simulink model "model_based_imp_ctrl_R2017b"  (Simulink 9.0)
settings: Solver=VariableStepAuto  StartTime=0.0  StopTime=60  FixedStep=0.00040  RelTol=1e-4  AbsTol=1e-7
values from neighbouring files (symbols this model uses):
  alpha = pi/180 * 13.6    (= 0.237364778271)    [IdealParameter.m]    (also in ParLuk11.m = deg2rad(13.6); Parameter.m = [-alpha_i;alpha_i;-alpha_i;alpha_i;-alpha_i;alpha_i]; ParameterIdeal.m = [-alpha_i;alpha_i;-alpha_i;alpha_i;-alpha_i;alpha_i]; ParameterVIVE.m = [alpha_i;-alpha_i;alpha_i;-alpha_i;alpha_i;-alpha_i])
  alpha_0 = alpha    (= 0.237364778271)    [IdealParameter.m]    (also in Parameter.m = alpha; ParameterIdeal.m = alpha*1.01; ParameterVIVE.m = alpha*1.01; ParameterVO.m = alpha*1.01)
  angular_noise = 0    [IdealParameter.m]    (also in Parameter.m = 0.5; ParameterIdeal.m; ParameterVIVE.m; ParameterVO.m)
  b = 1.1e-06    [IdealParameter.m]    (also in ParLuk11.m = 1.14e-07; Parameter.m = 8.944e-07; ParameterIdeal.m; ParameterVIVE.m)
  b_0 = b*1.15    (= 1.265e-06)    [IdealParameter.m]    (also in Parameter.m = 8.944e-07; ParameterIdeal.m; ParameterVIVE.m; ParameterVO.m)
  beta = 0    [IdealParameter.m]    (also in ParLuk11.m; Parameter.m = [beta_i; beta_i; beta_i; beta_i; beta_i; beta_i]; ParameterIdeal.m = [beta_i; beta_i; beta_i; beta_i; beta_i; beta_i]; ParameterVIVE.m = [beta_i; beta_i; beta_i; beta_i; beta_i; beta_i])
  beta_0 = beta    (= 0)    [IdealParameter.m]    (also in Parameter.m = beta; ParameterIdeal.m = beta*0.99; ParameterVIVE.m = beta*0.99; ParameterVO.m = beta*0.99)
  deltah = -0.0427    [Parameter.m]    (also in ParameterIdeal.m; ParameterVIVE.m = 0; ParameterVO.m; Parameter_old.m)
  deltah_0 = deltah    (= -0.0427)    [Parameter.m]    (also in ParameterIdeal.m = -0.041419; ParameterVIVE.m = 0; ParameterVO.m = -0.041419; Parameter_old.m = -0.041419)
  eta_rot = 50    [IdealParameter.m]    (also in Parameter.m = 2; ParameterIdeal.m = 20; ParameterVIVE.m = 5; ParameterVO.m = 2)
  g = 9.81    [IdealParameter.m]    (also in ParLuk11.m; Parameter.m; ParameterIdeal.m; ParameterVIVE.m)
  g_0 = g*0.99    (= 9.7119)    [IdealParameter.m]    (also in Parameter.m = 9.81; ParameterIdeal.m = 9.81; ParameterVIVE.m = 9.81; ParameterVO.m = 9.81)
  IB = [Ixx 0 0; 0 Iyy 0; 0 0 Izz]    [IdealParameter.m]    (also in ParLuk11.m; Parameter.m; ParameterIdeal.m; ParameterVIVE.m)
  IB_0 = IB*1.07    [IdealParameter.m]    (also in Parameter.m = IB; ParameterIdeal.m; ParameterVIVE.m; ParameterVO.m)
  Ip = [Ipx 0 0; 0 Ipy 0; 0 0 Ipz]    [Parameter.m]    (also in ParameterIdeal.m; ParameterVIVE.m; ParameterVO.m; Parameter_old.m)
  k = 5.6e-05    [IdealParameter.m]    (also in ParLuk11.m = 2.98e-06; Parameter.m = 4.472e-05; ParameterIdeal.m; ParameterVIVE.m = 5.13e-05)
  K_0 = Ts/(T_rotor_0+Ts)    (= 0.0384615384615)    [IdealParameter.m]    (also in Parameter.m = 0.230769230769; ParameterIdeal.m; ParameterVIVE.m = 0.0350877192982; ParameterVO.m = 0.214285714286)
  k_0 = k*1.16    (= 6.496e-05)    [IdealParameter.m]    (also in Parameter.m = 4.472e-05; ParameterIdeal.m; ParameterVIVE.m = 5.9508e-05; ParameterVO.m)
  K_d_star = 4*eye(3)    [Parameter.m]    (also in ParameterIdeal.m; ParameterVIVE.m; ParameterVO.m; Parameter_old.m)
  K_p_star = 50*eye(3)    [Parameter.m]    (also in ParameterIdeal.m; ParameterVIVE.m; ParameterVO.m; Parameter_old.m)
  L = 0.4    [IdealParameter.m]    (also in ParLuk11.m = 1; Parameter.m; ParameterIdeal.m; ParameterVIVE.m = 0.6)
  L_0 = L*1.02    (= 0.408)    [IdealParameter.m]    (also in Parameter.m = 0.4; ParameterIdeal.m; ParameterVIVE.m = 0.612; ParameterVO.m)
  lambda_rot = 10    [IdealParameter.m]    (also in Parameter.m = 3; ParameterIdeal.m; ParameterVIVE.m = 5; ParameterVO.m = 3)
  m = 1    [Controllability.m]    (also in IdealParameter.m = 2.5; ParLuk11.m = 0.6; Parameter.m = 4.85; ParameterIdeal.m = 4.85)
  m_0 = m*1.03    (= 2.575)    [IdealParameter.m]    (also in Parameter.m = 4.85; ParameterIdeal.m = 4.9955; ParameterVIVE.m = 4.52994; ParameterVO.m = 4.9955)
  M_rot = 50    [IdealParameter.m]    (also in Parameter.m = 6; ParameterIdeal.m = 15; ParameterVIVE.m = 1; ParameterVO.m = 6)
  M_star = m_0*eye(3)    [Parameter.m]    (also in ParameterIdeal.m; ParameterVIVE.m; ParameterVO.m; Parameter_old.m)
  mp = 0.05    [Parameter.m]    (also in ParameterIdeal.m; ParameterVIVE.m; ParameterVO.m; Parameter_old.m)
  omega_noise = 0    [IdealParameter.m]    (also in Parameter.m = sqrt(2)*angular_noise/Ts * pi/180; ParameterIdeal.m; ParameterVIVE.m; ParameterVO.m)
  p_noise = 0    [IdealParameter.m]    (also in Parameter.m = 0.001; ParameterIdeal.m; ParameterVIVE.m; ParameterVO.m)
  T_delay = 0    [IdealParameter.m]    (also in Parameter.m = 0.1; ParameterIdeal.m; ParameterVIVE.m = 0.04; ParameterVO.m = 0.1)
  T_rotor = 0.1    [IdealParameter.m]    (also in Parameter.m; ParameterIdeal.m; ParameterVIVE.m; ParameterVO.m)
  Ts = 1/250    (= 0.004)    [IdealParameter.m]    (also in Parameter.m = 0.03; ParameterIdeal.m; ParameterVIVE.m; ParameterVO.m = 0.03)
  v_noise = 0    [IdealParameter.m]    (also in Parameter.m = sqrt(2)*p_noise/Ts; ParameterIdeal.m; ParameterVIVE.m; ParameterVO.m)
  z_p_0 = T_rotor_0/(T_rotor_0+Ts)    (= 0.961538461538)    [IdealParameter.m]    (also in Parameter.m = 0.769230769231; ParameterIdeal.m; ParameterVIVE.m = 0.964912280702; ParameterVO.m = 0.785714285714)
undefined symbols (not defined in the file or in its folder): DiscIntNeverNeededParam, mm
libraries: simulink x7, vrlib x2, slctrlblks x1, dspinverses x1
(part 3 of 3)

== matlab function Motion Equations backup/MATLAB Function9 ==
  data: result output double; q input double; q_dot input double
function result = fcn(q,q_dot)

% q1=q(1);
% q2=q(2);
% q3=q(3);
% q4=q(4);
% w1=w(1);
% w2=w(2);
% w3=w(3);
% coder.extrinsic('mysyms');
% result = zeros(4,1);
% result = mysyms(w1,w2,w3,q1,q2,q3,q4);
% Ixx = 0.5;
% Iyy = Ixx;
% Izz = 2;
% result=[ (Iyy*q1(t)^3*w1(t)^2)/4 + (Izz*q1(t)^3*w2(t)^2)/4 + (Ixx*q1(t)*q2(t)^2*w1(t)^2)/8 + (Ixx*q1(t)*q2(t)^2*w3(t)^2)/8 + (Ixx*q1(t)*q3(t)^2*w2(t)^2)/2 + (Ixx*q1(t)*q4(t)^2*w1(t)^2)/8 - (Ixx*q2(t)^2*q3(t)*w1(t)^2)/8 + (Ixx*q2(t)^2*q3(t)*w2(t)^2)/4 + (Ixx*q1(t)*q4(t)^2*w3(t)^2)/8 - (Ixx*q3(t)*q4(t)^2*w1(t)^2)/8 - (Ixx*q2(t)^2*q3(t)*w3(t)^2)/8 + (Ixx*q3(t)*q4(t)^2*w2(t)^2)/4 - (Ixx*q3(t)*q4(t)^2*w3(t)^2)/8 + (Iyy*q1(t)*q2(t)^2*w2(t)^2)/8 + (Iyy*q1(t)*q3(t)^2*w1(t)^2)/4 + (Iyy*q1(t)*q4(t)^2*w2(t)^2)/8 - (Iyy*q2(t)^2*q3(t)*w2(t)^2)/8 - (Iyy*q3(t)*q4(t)^2*w2(t)^2)/8 + (Izz*q1(t)*q2(t)^2*w1(t)^2)/8 + (Izz*q1(t)*q2(t)^2*w3(t)^2)/8 - (Izz*q1(t)*q3(t)^2*w2(t)^2)/4 + (Izz*q1(t)*q4(t)^2*w1(t)^2)/8 + (Izz*q2(t)^2*q3(t)*w1(t)^2)/8 + (Izz*q1(t)*q4(t)^2*w3(t)^2)/8 + (Izz*q3(t)*q4(t)^2*w1(t)^2)/8 + (Izz*q2(t)^2*q3(t)*w3(t)^2)/8 + (Izz*q3(t)*q4(t)^2*w3(t)^2)/8 + (Ixx*q2(t)^3*w1(t)*w2(t))/8 - (Ixx*q2(t)^3*w2(t)*w3(t))/8 - (Ixx*q4(t)^3*w1(t)*w2(t))/8 - (Ixx*q4(t)^3*w2(t)*w3(t))/8 + (Iyy*q2(t)^3*w2(t)*w3(t))/8 + (Iyy*q4(t)^3*w2(t)*w3(t))/8 - (Ixx*q1(t)*q2(t)*q4(t)*w1(t)^2)/4 + (Ixx*q1(t)*q2(t)*q4(t)*w3(t)^2)/4 + (Ixx*q2(t)*q3(t)*q4(t)*w1(t)^2)/4 - (Ixx*q2(t)*q3(t)*q4(t)*w3(t)^2)/4 + (Iyy*q1(t)*q2(t)*q4(t)*w1(t)^2)/2 - (Iyy*q1(t)*q2(t)*q4(t)*w2(t)^2)/4 + (Iyy*q2(t)*q3(t)*q4(t)*w2(t)^2)/4 - (Izz*q1(t)*q2(t)*q4(t)*w1(t)^2)/4 + (Izz*q1(t)*q2(t)*q4(t)*w3(t)^2)/4 - (Izz*q2(t)*q3(t)*q4(t)*w1(t)^2)/4 + (Izz*q2(t)*q3(t)*q4(t)*w3(t)^2)/4 - (Ixx*q1(t)*q2(t)^2*w1(t)*w3(t))/4 - (Ixx*q2(t)*q3(t)^2*w1(t)*w2(t))/4 + (Ixx*q1(t)*q4(t)^2*w1(t)*w3(t))/4 + (Ixx*q2(t)*q4(t)^2*w1(t)*w2(t))/8 + (Ixx*q2(t)^2*q3(t)*w1(t)*w3(t))/4 - (Ixx*q2(t)^2*q4(t)*w1(t)*w2(t))/8 + (Ixx*q2(t)*q3(t)^2*w2(t)*w3(t))/4 + (Ixx*q3(t)^2*q4(t)*w1(t)*w2(t))/4 - (Ixx*q2(t)*q4(t)^2*w2(t)*w3(t))/8 - (Ixx*q3(t)*q4(t)^2*w1(t)*w3(t))/4 - (Ixx*q2(t)^2*q4(t)*w2(t)*w3(t))/8 + (Ixx*q3(t)^2*q4(t)*w2(t)*w3(t))/4 + (3*Iyy*q1(t)^2*q2(t)*w1(t)*w2(t))/8 + (Iyy*q1(t)*q2(t)^2*w1(t)*w3(t))/4 + (Iyy*q2(t)*q3(t)^2*w1(t)*w2(t))/8 - (3*Iyy*q1(t)^2*q4(t)*w1(t)*w2(t))/8 - (Iyy*q1(t)*q4(t)^2*w1(t)*w3(t))/4 - (Iyy*q2(t)*q4(t)^2*w1(t)*w2(t))/4 + (Iyy*q2(t)^2*q4(t)*w1(t)*w2(t))/4 - (Iyy*q3(t)^2*q4(t)*w1(t)*w2(t))/8 - (Iyy*q2(t)*q4(t)^2*w2(t)*w3(t))/8 - (Iyy*q2(t)^2*q4(t)*w2(t)*w3(t))/8 - (3*Izz*q1(t)^2*q2(t)*w1(t)*w2(t))/8 - (Izz*q1(t)*q2(t)^2*w1(t)*w3(t))/4 + (Izz*q2(t)*q3(t)^2*w1(t)*w2(t))/8 + (3*Izz*q1(t)^2*q2(t)*w2(t)*w3(t))/8 + (3*Izz*q1(t)^2*q4(t)*w1(t)*w2(t))/8 + (Izz*q1(t)*q4(t)^2*w1(t)*w3(t))/4 - (Izz*q2(t)^2*q3(t)*w1(t)*w3(t))/4 - (Izz*q2(t)*q3(t)^2*w2(t)*w3(t))/8 + (3*Izz*q1(t)^2*q4(t)*w2(t)*w3(t))/8 - (Izz*q3(t)^2*q4(t)*w1(t)*w2(t))/8 + (Izz*q3(t)*q4(t)^2*w1(t)*w3(t))/4 - (Izz*q3(t)^2*q4(t)*w2(t)*w3(t))/8 + (Ixx*q1(t)*q2(t)*q3(t)*w1(t)*w2(t))/2 - (Ixx*q1(t)*q2(t)*q3(t)*w2(t)*w3(t))/2 - (Ixx*q1(t)*q3(t)*q4(t)*w1(t)*w2(t))/2 - (Ixx*q1(t)*q3(t)*q4(t)*w2(t)*w3(t))/2 - (Iyy*q1(t)*q2(t)*q3(t)*w1(t)*w2(t))/4 + (Iyy*q1(t)*q3(t)*q4(t)*w1(t)*w2(t))/4 - (Izz*q1(t)*q2(t)*q3(t)*w1(t)*w2(t))/4 + (Izz*q1(t)*q2(t)*q3(t)*w2(t)*w3(t))/4 + (Izz*q1(t)*q3(t)*q4(t)*w1(t)*w2(t))/4 + (Izz*q1(t)*q3(t)*q4(t)*w2(t)*w3(t))/4, (Ixx*q2(t)^3*w2(t)^2)/4 + (Iyy*q2(t)^3*w3(t)^2)/4 + (Ixx*q1(t)^2*q2(t)*w1(t)^2)/8 + (Ixx*q2(t)*q3(t)^2*w1(t)^2)/8 + (Ixx*q1(t)^2*q2(t)*w3(t)^2)/8 - (Ixx*q1(t)^2*q4(t)*w1(t)^2)/8 + (Ixx*q2(t)*q3(t)^2*w3(t)^2)/8 + (Ixx*q2(t)*q4(t)^2*w2(t)^2)/4 + (Ixx*q1(t)^2*q4(t)*w3(t)^2)/8 - (Ixx*q3(t)^2*q4(t)*w1(t)^2)/8 + (Ixx*q3(t)^2*q4(t)*w3(t)^2)/8 + (Iyy*q1(t)^2*q2(t)*w2(t)^2)/8 + (Iyy*q1(t)^2*q4(t)*w1(t)^2)/4 + (Iyy*q2(t)*q3(t)^2*w2(t)^2)/8 + (Iyy*q2(t)*q4(t)^2*w1(t)^2)/2 - (Iyy*q1(t)^2*q4(t)*w2(t)^2)/8 + (Iyy*q3(t)^2*q4(t)*w1(t)^2)/4 - (Iyy*q2(t)*q4(t)^2*w3(t)^2)/4 - (Iyy*q3(t)^2*q4(t)*w2(t)^2)/8 + (Izz*q1(t)^2*q2(t)*w1(t)^2)/8 + (Izz*q2(t)*q3(t)^2*w1(t)^2)/8 + (Izz*q1(t)^2*q2(t)*w3(t)^2)/8 - (Izz*q1(t)^2*q4(t)*w1(t)^2)/8 + (Izz*q2(t)*q3(t)^2*w3(t)^2)/8 + (Izz*q1(t)^2*q4(t)*w3(t)^2)/8 - (Izz*q3(t)^2*q4(t)*w1(t)^2)/8 + (Izz*q3(t)^2*q4(t)*w3(t)^2)/8 + (Iyy*q1(t)^3*w1(t)*w2(t))/8 - (Iyy*q3(t)^3*w1(t)*w2(t))/8 - (Iyy*q4(t)^3*w1(t)*w3(t))/4 - (Izz*q1(t)^3*w1(t)*w2(t))/8 + (Izz*q1(t)^3*w2(t)*w3(t))/8 + (Izz*q3(t)^3*w1(t)*w2(t))/8 - (Izz*q3(t)^3*w2(t)*w3(t))/8 - (Ixx*q1(t)*q2(t)*q3(t)*w1(t)^2)/4 + (Ixx*q1(t)*q2(t)*q3(t)*w2(t)^2)/2 - (Ixx*q1(t)*q2(t)*q3(t)*w3(t)^2)/4 + (Ixx*q1(t)*q3(t)*q4(t)*w1(t)^2)/4 - (Ixx*q1(t)*q3(t)*q4(t)*w3(t)^2)/4 - (Iyy*q1(t)*q2(t)*q3(t)*w2(t)^2)/4 + (Iyy*q1(t)*q3(t)*q4(t)*w2(t)^2)/4 + (Izz*q1(t)*q2(t)*q3(t)*w1(t)^2)/4 + (Izz*q1(t)*q2(t)*q3(t)*w3(t)^2)/4 - (Izz*q1(t)*q3(t)*q4(t)*w1(t)^2)/4 + (Izz*q1(t)*q3(t)*q4(t)*w3(t)^2)/4 + (3*Ixx*q1(t)*q2(t)^2*w1(t)*w2(t))/8 - (Ixx*q1(t)*q3(t)^2*w1(t)*w2(t))/4 - (Ixx*q1(t)^2*q2(t)*w1(t)*w3(t))/4 + (Ixx*q1(t)^2*q3(t)*w1(t)*w2(t))/4 - (3*Ixx*q1(t)*q2(t)^2*w2(t)*w3(t))/8 + (Ixx*q1(t)*q4(t)^2*w1(t)*w2(t))/8 - (3*Ixx*q2(t)^2*q3(t)*w1(t)*w2(t))/8 + (Ixx*q1(t)*q3(t)^2*w2(t)*w3(t))/4 - (Ixx*q2(t)*q3(t)^2*w1(t)*w3(t))/4 - (Ixx*q1(t)^2*q3(t)*w2(t)*w3(t))/4 - (Ixx*q1(t)*q4(t)^2*w2(t)*w3(t))/8 - (Ixx*q3(t)*q4(t)^2*w1(t)*w2(t))/8 + (3*Ixx*q2(t)^2*q3(t)*w2(t)*w3(t))/8 + (Ixx*q3(t)*q4(t)^2*w2(t)*w3(t))/8 + (Iyy*q1(t)*q3(t)^2*w1(t)*w2(t))/8 + (Iyy*q1(t)^2*q2(t)*w1(t)*w3(t))/4 - (Iyy*q1(t)^2*q3(t)*w1(t)*w2(t))/8 + (3*Iyy*q1(t)*q2(t)^2*w2(t)*w3(t))/8 - (Iyy*q1(t)*q4(t)^2*w1(t)*w2(t))/4 + (Iyy*q2(t)*q3(t)^2*w1(t)*w3(t))/4 - (Iyy*q1(t)*q4(t)^2*w2(t)*w3(t))/8 + (Iyy*q3(t)*q4(t)^2*w1(t)*w2(t))/4 - (3*Iyy*q2(t)^2*q3(t)*w2(t)*w3(t))/8 + (3*Iyy*q2(t)^2*q4(t)*w1(t)*w3(t))/4 + (Iyy*q3(t)*q4(t)^2*w2(t)*w3(t))/8 + (Izz*q1(t)*q3(t)^2*w1(t)*w2(t))/8 - (Izz*q1(t)^2*q2(t)*w1(t)*w3(t))/4 - (Izz*q1(t)^2*q3(t)*w1(t)*w2(t))/8 - (Izz*q1(t)*q3(t)^2*w2(t)*w3(t))/8 - (Izz*q2(t)*q3(t)^2*w1(t)*w3(t))/4 + (Izz*q1(t)^2*q3(t)*w2(t)*w3(t))/8 + (Ixx*q1(t)*q2(t)*q3(t)*w1(t)*w3(t))/2 - (Ixx*q1(t)*q2(t)*q4(t)*w1(t)*w2(t))/4 - (Ixx*q1(t)*q2(t)*q4(t)*w2(t)*w3(t))/4 + (Ixx*q2(t)*q3(t)*q4(t)*w1(t)*w2(t))/4 + (Ixx*q2(t)*q3(t)*q4(t)*w2(t)*w3(t))/4 + (Iyy*q1(t)*q2(t)*q4(t)*w1(t)*w2(t))/2 - (Iyy*q1(t)*q2(t)*q4(t)*w2(t)*w3(t))/4 - (Iyy*q2(t)*q3(t)*q4(t)*w1(t)*w2(t))/2 + (Iyy*q2(t)*q3(t)*q4(t)*w2(t)*w3(t))/4 - (Izz*q1(t)*q2(t)*q3(t)*w1(t)*w3(t))/2, (Iyy*q3(t)^3*w1(t)^2)/4 + (Izz*q3(t)^3*w2(t)^2)/4 - (Ixx*q1(t)*q2(t)^2*w1(t)^2)/8 + (Ixx*q1(t)*q2(t)^2*w2(t)^2)/4 - (Ixx*q1(t)*q2(t)^2*w3(t)^2)/8 - (Ixx*q1(t)*q4(t)^2*w1(t)^2)/8 + (Ixx*q1(t)^2*q3(t)*w2(t)^2)/2 + (Ixx*q2(t)^2*q3(t)*w1(t)^2)/8 + (Ixx*q1(t)*q4(t)^2*w2(t)^2)/4 - (Ixx*q1(t)*q4(t)^2*w3(t)^2)/8 + (Ixx*q3(t)*q4(t)^2*w1(t)^2)/8 + (Ixx*q2(t)^2*q3(t)*w3(t)^2)/8 + (Ixx*q3(t)*q4(t)^2*w3(t)^2)/8 - (Iyy*q1(t)*q2(t)^2*w2(t)^2)/8 + (Iyy*q1(t)^2*q3(t)*w1(t)^2)/4 - (Iyy*q1(t)*q4(t)^2*w2(t)^2)/8 + (Iyy*q2(t)^2*q3(t)*w2(t)^2)/8 + (Iyy*q3(t)*q4(t)^2*w2(t)^2)/8 + (Izz*q1(t)*q2(t)^2*w1(t)^2)/8 + (Izz*q1(t)*q2(t)^2*w3(t)^2)/8 + (Izz*q1(t)*q4(t)^2*w1(t)^2)/8 - (Izz*q1(t)^2*q3(t)*w2(t)^2)/4 + (Izz*q2(t)^2*q3(t)*w1(t)^2)/8 + (Izz*q1(t)*q4(t)^2*w3(t)^2)/8 + (Izz*q3(t)*q4(t)^2*w1(t)^2)/8 + (Izz*q2(t)^2*q3(t)*w3(t)^2)/8 + (Izz*q3(t)*q4(t)^2*w3(t)^2)/8 - (Ixx*q2(t)^3*w1(t)*w2(t))/8 + (Ixx*q2(t)^3*w2(t)*w3(t))/8 + (Ixx*q4(t)^3*w1(t)*w2(t))/8 + (Ixx*q4(t)^3*w2(t)*w3(t))/8 - (Iyy*q2(t)^3*w2(t)*w3(t))/8- (Iyy*q4(t)^3*w2(t)*w3(t))/8 + (Ixx*q1(t)*q2(t)*q4(t)*w1(t)^2)/4 - (Ixx*q1(t)*q2(t)*q4(t)*w3(t)^2)/4 - (Ixx*q2(t)*q3(t)*q4(t)*w1(t)^2)/4 + (Ixx*q2(t)*q3(t)*q4(t)*w3(t)^2)/4 + (Iyy*q1(t)*q2(t)*q4(t)*w2(t)^2)/4 + (Iyy*q2(t)*q3(t)*q4(t)*w1(t)^2)/2 - (Iyy*q2(t)*q3(t)*q4(t)*w2(t)^2)/4 - (Izz*q1(t)*q2(t)*q4(t)*w1(t)^2)/4 + (Izz*q1(t)*q2(t)*q4(t)*w3(t)^2)/4 - (Izz*q2(t)*q3(t)*q4(t)*w1(t)^2)/4 + (Izz*q2(t)*q3(t)*q4(t)*w3(t)^2)/4 + (Ixx*q1(t)^2*q2(t)*w1(t)*w2(t))/4 + (Ixx*q1(t)*q2(t)^2*w1(t)*w3(t))/4 - (Ixx*q1(t)^2*q2(t)*w2(t)*w3(t))/4 - (Ixx*q1(t)^2*q4(t)*w1(t)*w2(t))/4 - (Ixx*q1(t)*q4(t)^2*w1(t)*w3(t))/4 - (Ixx*q2(t)*q4(t)^2*w1(t)*w2(t))/8 - (Ixx*q2(t)^2*q3(t)*w1(t)*w3(t))/4 + (Ixx*q2(t)^2*q4(t)*w1(t)*w2(t))/8 - (Ixx*q1(t)^2*q4(t)*w2(t)*w3(t))/4 + (Ixx*q2(t)*q4(t)^2*w2(t)*w3(t))/8 + (Ixx*q3(t)*q4(t)^2*w1(t)*w3(t))/4 + (Ixx*q2(t)^2*q4(t)*w2(t)*w3(t))/8 - (Iyy*q1(t)^2*q2(t)*w1(t)*w2(t))/8 - (3*Iyy*q2(t)*q3(t)^2*w1(t)*w2(t))/8 + (Iyy*q1(t)^2*q4(t)*w1(t)*w2(t))/8 + (Iyy*q2(t)*q4(t)^2*w1(t)*w2(t))/4 + (Iyy*q2(t)^2*q3(t)*w1(t)*w3(t))/4 - (Iyy*q2(t)^2*q4(t)*w1(t)*w2(t))/4 + (3*Iyy*q3(t)^2*q4(t)*w1(t)*w2(t))/8 + (Iyy*q2(t)*q4(t)^2*w2(t)*w3(t))/8 - (Iyy*q3(t)*q4(t)^2*w1(t)*w3(t))/4 + (Iyy*q2(t)^2*q4(t)*w2(t)*w3(t))/8 - (Izz*q1(t)^2*q2(t)*w1(t)*w2(t))/8 - (Izz*q1(t)*q2(t)^2*w1(t)*w3(t))/4 + (3*Izz*q2(t)*q3(t)^2*w1(t)*w2(t))/8 + (Izz*q1(t)^2*q2(t)*w2(t)*w3(t))/8 + (Izz*q1(t)^2*q4(t)*w1(t)*w2(t))/8 + (Izz*q1(t)*q4(t)^2*w1(t)*w3(t))/4 - (Izz*q2(t)^2*q3(t)*w1(t)*w3(t))/4 - (3*Izz*q2(t)*q3(t)^2*w2(t)*w3(t))/8 + (Izz*q1(t)^2*q4(t)*w2(t)*w3(t))/8 - (3*Izz*q3(t)^2*q4(t)*w1(t)*w2(t))/8 + (Izz*q3(t)*q4(t)^2*w1(t)*w3(t))/4 - (3*Izz*q3(t)^2*q4(t)*w2(t)*w3(t))/8 - (Ixx*q1(t)*q2(t)*q3(t)*w1(t)*w2(t))/2 + (Ixx*q1(t)*q2(t)*q3(t)*w2(t)*w3(t))/2 + (Ixx*q1(t)*q3(t)*q4(t)*w1(t)*w2(t))/2 + (Ixx*q1(t)*q3(t)*q4(t)*w2(t)*w3(t))/2 + (Iyy*q1(t)*q2(t)*q3(t)*w1(t)*w2(t))/4 - (Iyy*q1(t)*q3(t)*q4(t)*w1(t)*w2(t))/4 + (Izz*q1(t)*q2(t)*q3(t)*w1(t)*w2(t))/4 - (Izz*q1(t)*q2(t)*q3(t)*w2(t)*w3(t))/4 - (Izz*q1(t)*q3(t)*q4(t)*w1(t)*w2(t))/4 - (Izz*q1(t)*q3(t)*q4(t)*w2(t)*w3(t))/4, (Ixx*q4(t)^3*w2(t)^2)/4 + (Iyy*q4(t)^3*w3(t)^2)/4 - (Ixx*q1(t)^2*q2(t)*w1(t)^2)/8 - (Ixx*q2(t)*q3(t)^2*w1(t)^2)/8 + (Ixx*q1(t)^2*q2(t)*w3(t)^2)/8 + (Ixx*q1(t)^2*q4(t)*w1(t)^2)/8 + (Ixx*q2(t)*q3(t)^2*w3(t)^2)/8 + (Ixx*q1(t)^2*q4(t)*w3(t)^2)/8 + (Ixx*q2(t)^2*q4(t)*w2(t)^2)/4 + (Ixx*q3(t)^2*q4(t)*w1(t)^2)/8 + (Ixx*q3(t)^2*q4(t)*w3(t)^2)/8 + (Iyy*q1(t)^2*q2(t)*w1(t)^2)/4 - (Iyy*q1(t)^2*q2(t)*w2(t)^2)/8 + (Iyy*q2(t)*q3(t)^2*w1(t)^2)/4 - (Iyy*q2(t)*q3(t)^2*w2(t)^2)/8 + (Iyy*q1(t)^2*q4(t)*w2(t)^2)/8 + (Iyy*q2(t)^2*q4(t)*w1(t)^2)/2 - (Iyy*q2(t)^2*q4(t)*w3(t)^2)/4 + (Iyy*q3(t)^2*q4(t)*w2(t)^2)/8 - (Izz*q1(t)^2*q2(t)*w1(t)^2)/8 - (Izz*q2(t)*q3(t)^2*w1(t)^2)/8 + (Izz*q1(t)^2*q2(t)*w3(t)^2)/8 + (Izz*q1(t)^2*q4(t)*w1(t)^2)/8 + (Izz*q2(t)*q3(t)^2*w3(t)^2)/8 + (Izz*q1(t)^2*q4(t)*w3(t)^2)/8 + (Izz*q3(t)^2*q4(t)*w1(t)^2)/8 + (Izz*q3(t)^2*q4(t)*w3(t)^2)/8 - (Iyy*q1(t)^3*w1(t)*w2(t))/8 + (Iyy*q2(t)^3*w1(t)*w3(t))/4 + (Iyy*q3(t)^3*w1(t)*w2(t))/8 + (Izz*q1(t)^3*w1(t)*w2(t))/8 + (Izz*q1(t)^3*w2(t)*w3(t))/8 - (Izz*q3(t)^3*w1(t)*w2(t))/8 - (Izz*q3(t)^3*w2(t)*w3(t))/8 + (Ixx*q1(t)*q2(t)*q3(t)*w1(t)^2)/4 - (Ixx*q1(t)*q2(t)*q3(t)*w3(t)^2)/4 - (Ixx*q1(t)*q3(t)*q4(t)*w1(t)^2)/4 + (Ixx*q1(t)*q3(t)*q4(t)*w2(t)^2)/2 - (Ixx*q1(t)*q3(t)*q4(t)*w3(t)^2)/4 + (Iyy*q1(t)*q2(t)*q3(t)*w2(t)^2)/4 - (Iyy*q1(t)*q3(t)*q4(t)*w2(t)^2)/4 - (Izz*q1(t)*q2(t)*q3(t)*w1(t)^2)/4 + (Izz*q1(t)*q2(t)*q3(t)*w3(t)^2)/4 + (Izz*q1(t)*q3(t)*q4(t)*w1(t)^2)/4 + (Izz*q1(t)*q3(t)*q4(t)*w3(t)^2)/4 - (Ixx*q1(t)*q2(t)^2*w1(t)*w2(t))/8 + (Ixx*q1(t)*q3(t)^2*w1(t)*w2(t))/4 - (Ixx*q1(t)^2*q3(t)*w1(t)*w2(t))/4 - (Ixx*q1(t)*q2(t)^2*w2(t)*w3(t))/8 - (3*Ixx*q1(t)*q4(t)^2*w1(t)*w2(t))/8 + (Ixx*q2(t)^2*q3(t)*w1(t)*w2(t))/8 + (Ixx*q1(t)*q3(t)^2*w2(t)*w3(t))/4 - (Ixx*q1(t)^2*q3(t)*w2(t)*w3(t))/4 + (Ixx*q1(t)^2*q4(t)*w1(t)*w3(t))/4 - (3*Ixx*q1(t)*q4(t)^2*w2(t)*w3(t))/8 + (3*Ixx*q3(t)*q4(t)^2*w1(t)*w2(t))/8 + (Ixx*q2(t)^2*q3(t)*w2(t)*w3(t))/8 + (Ixx*q3(t)^2*q4(t)*w1(t)*w3(t))/4 + (3*Ixx*q3(t)*q4(t)^2*w2(t)*w3(t))/8 + (Iyy*q1(t)*q2(t)^2*w1(t)*w2(t))/4 - (Iyy*q1(t)*q3(t)^2*w1(t)*w2(t))/8 + (Iyy*q1(t)^2*q3(t)*w1(t)*w2(t))/8 - (Iyy*q1(t)*q2(t)^2*w2(t)*w3(t))/8 - (Iyy*q2(t)^2*q3(t)*w1(t)*w2(t))/4 - (Iyy*q1(t)^2*q4(t)*w1(t)*w3(t))/4 + (3*Iyy*q1(t)*q4(t)^2*w2(t)*w3(t))/8 - (3*Iyy*q2(t)*q4(t)^2*w1(t)*w3(t))/4 + (Iyy*q2(t)^2*q3(t)*w2(t)*w3(t))/8 - (Iyy*q3(t)^2*q4(t)*w1(t)*w3(t))/4 - (3*Iyy*q3(t)*q4(t)^2*w2(t)*w3(t))/8 - (Izz*q1(t)*q3(t)^2*w1(t)*w2(t))/8 + (Izz*q1(t)^2*q3(t)*w1(t)*w2(t))/8 - (Izz*q1(t)*q3(t)^2*w2(t)*w3(t))/8 + (Izz*q1(t)^2*q3(t)*w2(t)*w3(t))/8 + (Izz*q1(t)^2*q4(t)*w1(t)*w3(t))/4 + (Izz*q3(t)^2*q4(t)*w1(t)*w3(t))/4 + (Ixx*q1(t)*q2(t)*q4(t)*w1(t)*w2(t))/4 - (Ixx*q1(t)*q2(t)*q4(t)*w2(t)*w3(t))/4 - (Ixx*q1(t)*q3(t)*q4(t)*w1(t)*w3(t))/2 - (Ixx*q2(t)*q3(t)*q4(t)*w1(t)*w2(t))/4 + (Ixx*q2(t)*q3(t)*q4(t)*w2(t)*w3(t))/4 - (Iyy*q1(t)*q2(t)*q4(t)*w1(t)*w2(t))/2 - (Iyy*q1(t)*q2(t)*q4(t)*w2(t)*w3(t))/4 + (Iyy*q2(t)*q3(t)*q4(t)*w1(t)*w2(t))/2 + (Iyy*q2(t)*q3(t)*q4(t)*w2(t)*w3(t))/4 + (Izz*q1(t)*q3(t)*q4(t)*w1(t)*w3(t))/2]

% result=[ (w2*(((3*q1*q4)/8 + (q2*q3)/8)*((q1*w1)/2 + (q2*w2)/2 + (q3*w3)/2) + ((3*q1*q3)/8 - (q2*q4)/8)*((q2*w3)/2 - (q3*w2)/2 + (q4*w1)/2) + ((q1*w2)/2 - (q2*w1)/2 + (q4*w3)/2)*(q1^2/2 + q3^2/8 + q4^2/8) - (q1*q2*((q3*w1)/2 - (q1*w3)/2 + (q4*w2)/2))/2))/2 + (w1*(((3*q1*q4)/8 + (q2*q3)/8)*((q1*w2)/2 - (q2*w1)/2 + (q4*w3)/2) + ((q1*q3)/8 - (3*q2*q4)/8)*((q3*w1)/2 - (q1*w3)/2 + (q4*w2)/2) + ((q1*w1)/2 + (q2*w2)/2 + (q3*w3)/2)*(q1^2/8 + q2^2/8 + q4^2/2) + (q3*q4*((q2*w3)/2 - (q3*w2)/2 + (q4*w1)/2))/2))/2 - (w3*(((q1*q3)/8 - (3*q2*q4)/8)*((q1*w1)/2 + (q2*w2)/2 + (q3*w3)/2) - ((q1*q4)/8 + (3*q2*q3)/8)*((q2*w3)/2 - (q3*w2)/2 + (q4*w1)/2) + ((q3*w1)/2 - (q1*w3)/2 + (q4*w2)/2)*(q2^2/2 + q3^2/8 + q4^2/8) - (q1*q2*((q1*w2)/2 - (q2*w1)/2 + (q4*w3)/2))/2))/2 + ((q2*w3)/2 - (q3*w2)/2 + (q4*w1)/2)*((q1*((q2*w3)/2 - (q3*w2)/2 + (q4*w1)/2))/4 + (3*q3*((q1*w2)/2 - (q2*w1)/2 + (q4*w3)/2))/8 - (q4*((q3*w1)/2 - (q1*w3)/2 + (q4*w2)/2))/8 + (w2*((3*q1*q3)/8 - (q2*q4)/8))/2 + (w3*((q1*q4)/8 + (3*q2*q3)/8))/2 + (q3*q4*w1)/4) - ((q3*w1)/2 - (q1*w3)/2 + (q4*w2)/2)*((q2*((q1*w2)/2 - (q2*w1)/2 + (q4*w3)/2))/2 - (q3*((q1*w1)/2 + (q2*w2)/2 + (q3*w3)/2))/8 + (q4*((q2*w3)/2 - (q3*w2)/2 + (q4*w1)/2))/8 - (w1*((q1*q3)/8 - (3*q2*q4)/8))/2 + (w3*(q2^2/2 + q3^2/8 + q4^2/8))/2 + (q1*q2*w2)/4) + ((q1*w1)/2 + (q2*w2)/2 + (q3*w3)/2)*((q1*((q1*w1)/2 + (q2*w2)/2 + (q3*w3)/2))/4 + (q3*((q3*w1)/2 - (q1*w3)/2 + (q4*w2)/2))/8 + (3*q4*((q1*w2)/2 - (q2*w1)/2 + (q4*w3)/2))/8 + (w2*((3*q1*q4)/8 + (q2*q3)/8))/2 - (w3*((q1*q3)/8 - (3*q2*q4)/8))/2 + (w1*(q1^2/8 + q2^2/8 + q4^2/2))/2) + ((q1*w2)/2 - (q2*w1)/2 + (q4*w3)/2)*(q1*((q1*w2)/2 - (q2*w1)/2 + (q4*w3)/2) - (q2*((q3*w1)/2 - (q1*w3)/2 + (q4*w2)/2))/2 + (3*q4*((q1*w1)/2 + (q2*w2)/2 + (q3*w3)/2))/8 + (3*q3*((q2*w3)/2 - (q3*w2)/2 + (q4*w1)/2))/8 + (w1*((3*q1*q4)/8 + (q2*q3)/8))/2 + (w2*(q1^2/2 + q3^2/8 + q4^2/8))/2 + (q1*q2*w3)/4), (w2*(((3*q1*q4)/8 + (q2*q3)/8)*((q1*w2)/2 - (q2*w1)/2 + (q4*w3)/2) + ((q1*q3)/8 - (3*q2*q4)/8)*((q3*w1)/2 - (q1*w3)/2 + (q4*w2)/2) + ((q1*w1)/2 + (q2*w2)/2 + (q3*w3)/2)*(q1^2/8 + q2^2/8 + q4^2/2) + (q3*q4*((q2*w3)/2 - (q3*w2)/2 + (q4*w1)/2))/2))/2 - (w1*(((3*q1*q4)/8 + (q2*q3)/8)*((q1*w1)/2 + (q2*w2)/2 + (q3*w3)/2) + ((3*q1*q3)/8 - (q2*q4)/8)*((q2*w3)/2 - (q3*w2)/2 + (q4*w1)/2) + ((q1*w2)/2 - (q2*w1)/2 + (q4*w3)/2)*(q1^2/2 + q3^2/8 + q4^2/8) - (q1*q2*((q3*w1)/2 - (q1*w3)/2 + (q4*w2)/2))/2))/2 + (w3*(((3*q1*q3)/8 - (q2*q4)/8)*((q1*w2)/2 - (q2*w1)/2 + (q4*w3)/2) - ((q1*q4)/8 + (3*q2*q3)/8)*((q3*w1)/2 - (q1*w3)/2 + (q4*w2)/2) + ((q2*w3)/2 - (q3*w2)/2 + (q4*w1)/2)*(q1^2/8 + q2^2/8 + q3^2/2) + (q3*q4*((q1*w1)/2 + (q2*w2)/2 + (q3*w3)/2))/2))/2 - ((q3*w1)/2 - (q1*w3)/2 + (q4*w2)/2)*((q1*((q1*w2)/2 - (q2*w1)/2 + (q4*w3)/2))/2 - q2*((q3*w1)/2 - (q1*w3)/2 + (q4*w2)/2) + (3*q4*((q1*w1)/2 + (q2*w2)/2 + (q3*w3)/2))/8 + (3*q3*((q2*w3)/2 - (q3*w2)/2 + (q4*w1)/2))/8 - (w2*((q1*q3)/8 - (3*q2*q4)/8))/2 + (w3*((q1*q4)/8 + (3*q2*q3)/8))/2 - (q1*q2*w1)/4) + ((q1*w1)/2 + (q2*w2)/2 + (q3*w3)/2)*((q2*((q1*w1)/2 + (q2*w2)/2 + (q3*w3)/2))/4 + (q3*((q1*w2)/2 - (q2*w1)/2 + (q4*w3)/2))/8 - (3*q4*((q3*w1)/2 - (q1*w3)/2 + (q4*w2)/2))/8 - (w1*((3*q1*q4)/8 + (q2*q3)/8))/2 + (w2*(q1^2/8 + q2^2/8 + q4^2/2))/2 + (q3*q4*w3)/4) + ((q2*w3)/2 - (q3*w2)/2 + (q4*w1)/2)*((q2*((q2*w3)/2 - (q3*w2)/2 + (q4*w1)/2))/4 - (3*q3*((q3*w1)/2 - (q1*w3)/2 + (q4*w2)/2))/8 - (q4*((q1*w2)/2 - (q2*w1)/2 + (q4*w3)/2))/8 - (w1*((3*q1*q3)/8 - (q2*q4)/8))/2 + (w3*(q1^2/8 + q2^2/8 + q3^2/2))/2 + (q3*q4*w2)/4) - ((q1*w2)/2 - (q2*w1)/2 + (q4*w3)/2)*((q1*((q3*w1)/2 - (q1*w3)/2 + (q4*w2)/2))/2 - (q3*((q1*w1)/2 + (q2*w2)/2 + (q3*w3)/2))/8 + (q4*((q2*w3)/2 - (q3*w2)/2 + (q4*w1)/2))/8 - (w2*((3*q1*q4)/8 + (q2*q3)/8))/2 - (w3*((3*q1*q3)/8 - (q2*q4)/8))/2 + (w1*(q1^2/2 + q3^2/8 + q4^2/8))/2), (w1*(((q1*q3)/8 - (3*q2*q4)/8)*((q1*w1)/2 + (q2*w2)/2 + (q3*w3)/2) - ((q1*q4)/8 + (3*q2*q3)/8)*((q2*w3)/2 - (q3*w2)/2 + (q4*w1)/2) + ((q3*w1)/2 - (q1*w3)/2 + (q4*w2)/2)*(q2^2/2 + q3^2/8 + q4^2/8) - (q1*q2*((q1*w2)/2 - (q2*w1)/2 + (q4*w3)/2))/2))/2 - (w2*(((3*q1*q3)/8 - (q2*q4)/8)*((q1*w2)/2 - (q2*w1)/2 + (q4*w3)/2) - ((q1*q4)/8 + (3*q2*q3)/8)*((q3*w1)/2 - (q1*w3)/2 + (q4*w2)/2) + ((q2*w3)/2 - (q3*w2)/2 + (q4*w1)/2)*(q1^2/8 + q2^2/8 + q3^2/2) + (q3*q4*((q1*w1)/2 + (q2*w2)/2 + (q3*w3)/2))/2))/2 + (w3*(((3*q1*q4)/8 + (q2*q3)/8)*((q1*w2)/2 - (q2*w1)/2 + (q4*w3)/2) + ((q1*q3)/8 - (3*q2*q4)/8)*((q3*w1)/2 - (q1*w3)/2 + (q4*w2)/2) + ((q1*w1)/2 + (q2*w2)/2 + (q3*w3)/2)*(q1^2/8 + q2^2/8 + q4^2/2) + (q3*q4*((q2*w3)/2 - (q3*w2)/2 + (q4*w1)/2))/2))/2 + ((q1*w2)/2 - (q2*w1)/2 + (q4*w3)/2)*((q2*((q1*w1)/2 + (q2*w2)/2 + (q3*w3)/2))/8 + (3*q1*((q2*w3)/2 - (q3*w2)/2 + (q4*w1)/2))/8 + (q3*((q1*w2)/2 - (q2*w1)/2 + (q4*w3)/2))/4 - (w2*((3*q1*q3)/8 - (q2*q4)/8))/2 + (w3*((3*q1*q4)/8 + (q2*q3)/8))/2 - (q1*q2*w1)/4) + ((q1*w1)/2 + (q2*w2)/2 + (q3*w3)/2)*((q1*((q3*w1)/2 - (q1*w3)/2 + (q4*w2)/2))/8 + (q2*((q1*w2)/2 - (q2*w1)/2 + (q4*w3)/2))/8 + (q4*((q2*w3)/2 - (q3*w2)/2 + (q4*w1)/2))/2 + (w1*((q1*q3)/8 - (3*q2*q4)/8))/2 + (w3*(q1^2/8 + q2^2/8 + q4^2/2))/2 - (q3*q4*w2)/4) + ((q3*w1)/2 - (q1*w3)/2 + (q4*w2)/2)*((q1*((q1*w1)/2 + (q2*w2)/2 + (q3*w3)/2))/8 - (3*q2*((q2*w3)/2 - (q3*w2)/2 + (q4*w1)/2))/8 + (q3*((q3*w1)/2 - (q1*w3)/2 + (q4*w2)/2))/4 + (w2*((q1*q4)/8 + (3*q2*q3)/8))/2 + (w3*((q1*q3)/8 - (3*q2*q4)/8))/2 + (w1*(q2^2/2 + q3^2/8 + q4^2/8))/2) + ((q2*w3)/2 - (q3*w2)/2 + (q4*w1)/2)*((3*q1*((q1*w2)/2 - (q2*w1)/2 + (q4*w3)/2))/8 - (3*q2*((q3*w1)/2 - (q1*w3)/2 + (q4*w2)/2))/8 + (q4*((q1*w1)/2 + (q2*w2)/2 + (q3*w3)/2))/2 + q3*((q2*w3)/2 - (q3*w2)/2 + (q4*w1)/2) - (w1*((q1*q4)/8 + (3*q2*q3)/8))/2 - (w2*(q1^2/8 + q2^2/8 + q3^2/2))/2 + (q3*q4*w3)/4), (w3*(((3*q1*q4)/8 + (q2*q3)/8)*((q1*w1)/2 + (q2*w2)/2 + (q3*w3)/2) + ((3*q1*q3)/8 - (q2*q4)/8)*((q2*w3)/2 - (q3*w2)/2 + (q4*w1)/2) + ((q1*w2)/2 - (q2*w1)/2 + (q4*w3)/2)*(q1^2/2 + q3^2/8 + q4^2/8) - (q1*q2*((q3*w1)/2 - (q1*w3)/2 + (q4*w2)/2))/2))/2 + (w1*(((3*q1*q3)/8 - (q2*q4)/8)*((q1*w2)/2 - (q2*w1)/2 + (q4*w3)/2) - ((q1*q4)/8 + (3*q2*q3)/8)*((q3*w1)/2 - (q1*w3)/2 + (q4*w2)/2) + ((q2*w3)/2 - (q3*w2)/2 + (q4*w1)/2)*(q1^2/8 + q2^2/8 + q3^2/2) + (q3*q4*((q1*w1)/2 + (q2*w2)/2 + (q3*w3)/2))/2))/2 + (w2*(((q1*q3)/8 - (3*q2*q4)/8)*((q1*w1)/2 + (q2*w2)/2 + (q3*w3)/2) - ((q1*q4)/8 + (3*q2*q3)/8)*((q2*w3)/2 - (q3*w2)/2 + (q4*w1)/2) + ((q3*w1)/2 - (q1*w3)/2 + (q4*w2)/2)*(q2^2/2 + q3^2/8 + q4^2/8) - (q1*q2*((q1*w2)/2 - (q2*w1)/2 + (q4*w3)/2))/2))/2 + ((q1*w1)/2 + (q2*w2)/2 + (q3*w3)/2)*((3*q1*((q1*w2)/2 - (q2*w1)/2 + (q4*w3)/2))/8 - (3*q2*((q3*w1)/2 - (q1*w3)/2 + (q4*w2)/2))/8 + q4*((q1*w1)/2 + (q2*w2)/2 + (q3*w3)/2) + (q3*((q2*w3)/2 - (q3*w2)/2 + (q4*w1)/2))/2 + (w2*((q1*q3)/8 - (3*q2*q4)/8))/2 + (w3*((3*q1*q4)/8 + (q2*q3)/8))/2 + (q3*q4*w1)/4) + ((q1*w2)/2 - (q2*w1)/2 + (q4*w3)/2)*((3*q1*((q1*w1)/2 + (q2*w2)/2 + (q3*w3)/2))/8 - (q2*((q2*w3)/2 - (q3*w2)/2 + (q4*w1)/2))/8 + (q4*((q1*w2)/2 - (q2*w1)/2 + (q4*w3)/2))/4 + (w1*((3*q1*q3)/8 - (q2*q4)/8))/2 + (w3*(q1^2/2 + q3^2/8 + q4^2/8))/2 - (q1*q2*w2)/4) - ((q3*w1)/2 - (q1*w3)/2 + (q4*w2)/2)*((3*q2*((q1*w1)/2 + (q2*w2)/2 + (q3*w3)/2))/8 + (q1*((q2*w3)/2 - (q3*w2)/2 + (q4*w1)/2))/8 - (q4*((q3*w1)/2 - (q1*w3)/2 + (q4*w2)/2))/4 + (w1*((q1*q4)/8 + (3*q2*q3)/8))/2 - (w2*(q2^2/2 + q3^2/8 + q4^2/8))/2 + (q1*q2*w3)/4) - ((q2*w3)/2 - (q3*w2)/2 + (q4*w1)/2)*((q1*((q3*w1)/2 - (q1*w3)/2 + (q4*w2)/2))/8 + (q2*((q1*w2)/2 - (q2*w1)/2 + (q4*w3)/2))/8 - (q3*((q1*w1)/2 + (q2*w2)/2 + (q3*w3)/2))/2 + (w2*((q1*q4)/8 + (3*q2*q3)/8))/2 - (w3*((3*q1*q3)/8 - (q2*q4)/8))/2 - (w1*(q1^2/8 + q2^2/8 + q3^2/2))/2)].';
 %result=functionalDerivative(q_dot.'*J*q_dot,q);
%result=[ (Iyy*q(1)^3*w(1)^2)/4 + (Izz*q(1)^3*w(2)^2)/4 + (Ixx*q(1)*q(2)^2*w(1)^2)/8 + (Ixx*q(1)*q(2)^2*w(3)^2)/8 + (Ixx*q(1)*q(3)^2*w(2)^2)/2 + (Ixx*q(1)*q(4)^2*w(1)^2)/8 - (Ixx*q(2)^2*q(3)*w(1)^2)/8 + (Ixx*q(2)^2*q(3)*w(2)^2)/4 + (Ixx*q(1)*q(4)^2*w(3)^2)/8 - (Ixx*q(3)*q(4)^2*w(1)^2)/8 - (Ixx*q(2)^2*q(3)*w(3)^2)/8 + (Ixx*q(3)*q(4)^2*w(2)^2)/4 - (Ixx*q(3)*q(4)^2*w(3)^2)/8 + (Iyy*q(1)*q(2)^2*w(2)^2)/8 + (Iyy*q(1)*q(3)^2*w(1)^2)/4 + (Iyy*q(1)*q(4)^2*w(2)^2)/8 - (Iyy*q(2)^2*q(3)*w3(2)^2)/8 - (Iyy*q(3)*q(4)^2*w(2)^2)/8 + (Izz*q1(t)*q2(t)^2*w1(t)^2)/8 + (Izz*q1(t)*q2(t)^2*w3(t)^2)/8 - (Izz*q1(t)*q3(t)^2*w2(t)^2)/4 + (Izz*q1(t)*q4(t)^2*w1(t)^2)/8 + (Izz*q2(t)^2*q3(t)*w1(t)^2)/8 + (Izz*q1(t)*q4(t)^2*w3(t)^2)/8 + (Izz*q3(t)*q4(t)^2*w1(t)^2)/8 + (Izz*q2(t)^2*q3(t)*w3(t)^2)/8 + (Izz*q3(t)*q4(t)^2*w3(t)^2)/8 + (Ixx*q2(t)^3*w1(t)*w2(t))/8 - (Ixx*q2(t)^3*w2(t)*w3(t))/8 - (Ixx*q4(t)^3*w1(t)*w2(t))/8 - (Ixx*q4(t)^3*w2(t)*w3(t))/8 + (Iyy*q2(t)^3*w2(t)*w3(t))/8\\\r\n + (Iyy*q4(t)^3*w2(t)*w3(t))/8 - (Ixx*q1(t)*q2(t)*q4(t)*w1(t)^2)/4 + (Ixx*q1(t)*q2(t)*q4(t)*w3(t)^2)/4 + (Ixx*q2(t)*q3(t)*q4(t)*w1(t)^2)/4 - (Ixx*q2(t)*q3(t)*q4(t)*w3(t)^2)/4 + (Iyy*q1(t)*q2(t)*q4(t)*w1(t)^2)/2 - (Iyy*q1(t)*q2(t)*q4(t)*w2(t)^2)/4 + (Iyy*q2(t)*q3(t)*q4(t)*w2(t)^2)/4 - (Izz*q1(t)*q2(t)*q4(t)*w1(t)^2)/4 + (Izz*q1(t)*q2(t)*q4(t)*w3(t)^2)/4 - (Izz*q2(t)*q3(t)*q4(t)*w1(t)^2)/4 + (Izz*q2(t)*q3(t)*q4(t)*w3(t)^2)/4 - (Ixx*q1(t)*q2(t)^2*w1(t)*w3(t))/4 - (Ixx*q2(t)*q3(t)^2*w1(t)*w2(t))/4 + (Ixx*q1(t)*q4(t)^2*w1(t)*w3(t))/4 + (Ixx*q2(t)*q4(t)^2*w1(t)*w2(t))/8 + (Ixx*q2(t)^2*q3(t)*w1(t)*w3(t))/4 - (Ixx*q2(t)^2*q4(t)*w1(t)*w2(t))/8 + (Ixx*q2(t)*q3(t)^2*w2(t)*w3(t))/4 + (Ixx*q3(t)^2*q4(t)*w1(t)*w2(t))/4 - (Ixx*q2(t)*q4(t)^2*w2(t)*w3(t))/8 - (Ixx*q3(t)*q4(t)^2*w1(t)*w3(t))/4 - (Ixx*q2(t)^2*q4(t)*w2(t)*w3(t))/8 + (Ixx*q3(t)^2*q4(t)*w2(t)*w3(t))/4 + (3*Iyy*q1(t)^2*q2(t)*w1(t)*w2(t))/8 + (Iyy*q1(t)*q2(t)^2*w1(t)*w3(t))/4 + (Iyy*q2(t)*q3(t)^2*w1(t)*w2(t))/8 - (3*Iyy*q1(t)^2*q4(t)*w1(t)*w\\\r\n2(t))/8 - (Iyy*q1(t)*q4(t)^2*w1(t)*w3(t))/4 - (Iyy*q2(t)*q4(t)^2*w1(t)*w2(t))/4 + (Iyy*q2(t)^2*q4(t)*w1(t)*w2(t))/4 - (Iyy*q3(t)^2*q4(t)*w1(t)*w2(t))/8 - (Iyy*q2(t)*q4(t)^2*w2(t)*w3(t))/8 - (Iyy*q2(t)^2*q4(t)*w2(t)*w3(t))/8 - (3*Izz*q1(t)^2*q2(t)*w1(t)*w2(t))/8 - (Izz*q1(t)*q2(t)^2*w1(t)*w3(t))/4 + (Izz*q2(t)*q3(t)^2*w1(t)*w2(t))/8 + (3*Izz*q1(t)^2*q2(t)*w2(t)*w3(t))/8 + (3*Izz*q1(t)^2*q4(t)*w1(t)*w2(t))/8 + (Izz*q1(t)*q4(t)^2*w1(t)*w3(t))/4 - (Izz*q2(t)^2*q3(t)*w1(t)*w3(t))/4 - (Izz*q2(t)*q3(t)^2*w2(t)*w3(t))/8 + (3*Izz*q1(t)^2*q4(t)*w2(t)*w3(t))/8 - (Izz*q3(t)^2*q4(t)*w1(t)*w2(t))/8 + (Izz*q3(t)*q4(t)^2*w1(t)*w3(t))/4 - (Izz*q3(t)^2*q4(t)*w2(t)*w3(t))/8 + (Ixx*q1(t)*q2(t)*q3(t)*w1(t)*w2(t))/2 - (Ixx*q1(t)*q2(t)*q3(t)*w2(t)*w3(t))/2 - (Ixx*q1(t)*q3(t)*q4(t)*w1(t)*w2(t))/2 - (Ixx*q1(t)*q3(t)*q4(t)*w2(t)*w3(t))/2 - (Iyy*q1(t)*q2(t)*q3(t)*w1(t)*w2(t))/4 + (Iyy*q1(t)*q3(t)*q4(t)*w1(t)*w2(t))/4 - (Izz*q1(t)*q2(t)*q3(t)*w1(t)*w2(t))/4 + (Izz*q1(t)*q2(t)*q3(t)*w2(t)*w3(t))/4 + (Izz*q1(t)*q3\\\r\n(t)*q4(t)*w1(t)*w2(t))/4 + (Izz*q1(t)*q3(t)*q4(t)*w2(t)*w3(t))/4, (Ixx*q2(t)^3*w2(t)^2)/4 + (Iyy*q2(t)^3*w3(t)^2)/4 + (Ixx*q1(t)^2*q2(t)*w1(t)^2)/8 + (Ixx*q2(t)*q3(t)^2*w1(t)^2)/8 + (Ixx*q1(t)^2*q2(t)*w3(t)^2)/8 - (Ixx*q1(t)^2*q4(t)*w1(t)^2)/8 + (Ixx*q2(t)*q3(t)^2*w3(t)^2)/8 + (Ixx*q2(t)*q4(t)^2*w2(t)^2)/4 + (Ixx*q1(t)^2*q4(t)*w3(t)^2)/8 - (Ixx*q3(t)^2*q4(t)*w1(t)^2)/8 + (Ixx*q3(t)^2*q4(t)*w3(t)^2)/8 + (Iyy*q1(t)^2*q2(t)*w2(t)^2)/8 + (Iyy*q1(t)^2*q4(t)*w1(t)^2)/4 + (Iyy*q2(t)*q3(t)^2*w2(t)^2)/8 + (Iyy*q2(t)*q4(t)^2*w1(t)^2)/2 - (Iyy*q1(t)^2*q4(t)*w2(t)^2)/8 + (Iyy*q3(t)^2*q4(t)*w1(t)^2)/4 - (Iyy*q2(t)*q4(t)^2*w3(t)^2)/4 - (Iyy*q3(t)^2*q4(t)*w2(t)^2)/8 + (Izz*q1(t)^2*q2(t)*w1(t)^2)/8 + (Izz*q2(t)*q3(t)^2*w1(t)^2)/8 + (Izz*q1(t)^2*q2(t)*w3(t)^2)/8 - (Izz*q1(t)^2*q4(t)*w1(t)^2)/8 + (Izz*q2(t)*q3(t)^2*w3(t)^2)/8 + (Izz*q1(t)^2*q4(t)*w3(t)^2)/8 - (Izz*q3(t)^2*q4(t)*w1(t)^2)/8 + (Izz*q3(t)^2*q4(t)*w3(t)^2)/8 + (Iyy*q1(t)^3*w1(t)*w2(t))/8 - (Iyy*q3(t)^3*w1(t)*w2(t))/8 - (Iyy*q4(t)^3*w1(t)*w3(t))/4 - (Izz*q1(t)^3*w1(t)*w2(t))/8 + (Izz*q1(t)^3*w2(t)*w3(t))/8\\\r\n + (Izz*q3(t)^3*w1(t)*w2(t))/8 - (Izz*q3(t)^3*w2(t)*w3(t))/8 - (Ixx*q1(t)*q2(t)*q3(t)*w1(t)^2)/4 + (Ixx*q1(t)*q2(t)*q3(t)*w2(t)^2)/2 - (Ixx*q1(t)*q2(t)*q3(t)*w3(t)^2)/4 + (Ixx*q1(t)*q3(t)*q4(t)*w1(t)^2)/4 - (Ixx*q1(t)*q3(t)*q4(t)*w3(t)^2)/4 - (Iyy*q1(t)*q2(t)*q3(t)*w2(t)^2)/4 + (Iyy*q1(t)*q3(t)*q4(t)*w2(t)^2)/4 + (Izz*q1(t)*q2(t)*q3(t)*w1(t)^2)/4 + (Izz*q1(t)*q2(t)*q3(t)*w3(t)^2)/4 - (Izz*q1(t)*q3(t)*q4(t)*w1(t)^2)/4 + (Izz*q1(t)*q3(t)*q4(t)*w3(t)^2)/4 + (3*Ixx*q1(t)*q2(t)^2*w1(t)*w2(t))/8 - (Ixx*q1(t)*q3(t)^2*w1(t)*w2(t))/4 - (Ixx*q1(t)^2*q2(t)*w1(t)*w3(t))/4 + (Ixx*q1(t)^2*q3(t)*w1(t)*w2(t))/4 - (3*Ixx*q1(t)*q2(t)^2*w2(t)*w3(t))/8 + (Ixx*q1(t)*q4(t)^2*w1(t)*w2(t))/8 - (3*Ixx*q2(t)^2*q3(t)*w1(t)*w2(t))/8 + (Ixx*q1(t)*q3(t)^2*w2(t)*w3(t))/4 - (Ixx*q2(t)*q3(t)^2*w1(t)*w3(t))/4 - (Ixx*q1(t)^2*q3(t)*w2(t)*w3(t))/4 - (Ixx*q1(t)*q4(t)^2*w2(t)*w3(t))/8 - (Ixx*q3(t)*q4(t)^2*w1(t)*w2(t))/8 + (3*Ixx*q2(t)^2*q3(t)*w2(t)*w3(t))/8 + (Ixx*q3(t)*q4(t)^2*w2(t)*w3(t))/8 + (Iyy*q1(t)*q3(t)^2*w1(t)*w2(\\\r\nt))/8 + (Iyy*q1(t)^2*q2(t)*w1(t)*w3(t))/4 - (Iyy*q1(t)^2*q3(t)*w1(t)*w2(t))/8 + (3*Iyy*q1(t)*q2(t)^2*w2(t)*w3(t))/8 - (Iyy*q1(t)*q4(t)^2*w1(t)*w2(t))/4 + (Iyy*q2(t)*q3(t)^2*w1(t)*w3(t))/4 - (Iyy*q1(t)*q4(t)^2*w2(t)*w3(t))/8 + (Iyy*q3(t)*q4(t)^2*w1(t)*w2(t))/4 - (3*Iyy*q2(t)^2*q3(t)*w2(t)*w3(t))/8 + (3*Iyy*q2(t)^2*q4(t)*w1(t)*w3(t))/4 + (Iyy*q3(t)*q4(t)^2*w2(t)*w3(t))/8 + (Izz*q1(t)*q3(t)^2*w1(t)*w2(t))/8 - (Izz*q1(t)^2*q2(t)*w1(t)*w3(t))/4 - (Izz*q1(t)^2*q3(t)*w1(t)*w2(t))/8 - (Izz*q1(t)*q3(t)^2*w2(t)*w3(t))/8 - (Izz*q2(t)*q3(t)^2*w1(t)*w3(t))/4 + (Izz*q1(t)^2*q3(t)*w2(t)*w3(t))/8 + (Ixx*q1(t)*q2(t)*q3(t)*w1(t)*w3(t))/2 - (Ixx*q1(t)*q2(t)*q4(t)*w1(t)*w2(t))/4 - (Ixx*q1(t)*q2(t)*q4(t)*w2(t)*w3(t))/4 + (Ixx*q2(t)*q3(t)*q4(t)*w1(t)*w2(t))/4 + (Ixx*q2(t)*q3(t)*q4(t)*w2(t)*w3(t))/4 + (Iyy*q1(t)*q2(t)*q4(t)*w1(t)*w2(t))/2 - (Iyy*q1(t)*q2(t)*q4(t)*w2(t)*w3(t))/4 - (Iyy*q2(t)*q3(t)*q4(t)*w1(t)*w2(t))/2 + (Iyy*q2(t)*q3(t)*q4(t)*w2(t)*w3(t))/4 - (Izz*q1(t)*q2(t)*q3(t)*w1(t)*w3(t))/2, (Iyy*q3(t)^3*w1(t)^2)/4 + (Izz*q3(t)^3*w2(t)^2)/4 - (Ixx*q1(t)*q2(t)^2*w1(t)^2)/8 + (Ixx*q1(t)*q2(t)^2*w2(t)^2)/4 - (Ixx*q1(t)*q2(t)^2*w3(t)^2)/8 - (Ixx*q1(t)*q4(t)^2*w1(t)^2)/8 + (Ixx*q1(t)^2*q3(t)*w2(t)^2)/2 + (Ixx*q2(t)^2*q3(t)*w1(t)^2)/8 + (Ixx*q1(t)*q4(t)^2*w2(t)^2)/4 - (Ixx*q1(t)*q4(t)^2*w3(t)^2)/8 + (Ixx*q3(t)*q4(t)^2*w1(t)^2)/8 + (Ixx*q2(t)^2*q3(t)*w3(t)^2)/8 + (Ixx*q3(t)*q4(t)^2*w3(t)^2)/8 - (Iyy*q1(t)*q2(t)^2*w2(t)^2)/8 + (Iyy*q1(t)^2*q3(t)*w1(t)^2)/4 - (Iyy*q1(t)*q4(t)^2*w2(t)^2)/8 + (Iyy*q2(t)^2*q3(t)*w2(t)^2)/8 + (Iyy*q3(t)*q4(t)^2*w2(t)^2)/8 + (Izz*q1(t)*q2(t)^2*w1(t)^2)/8 + (Izz*q1(t)*q2(t)^2*w3(t)^2)/8 + (Izz*q1(t)*q4(t)^2*w1(t)^2)/8 - (Izz*q1(t)^2*q3(t)*w2(t)^2)/4 + (Izz*q2(t)^2*q3(t)*w1(t)^2)/8 + (Izz*q1(t)*q4(t)^2*w3(t)^2)/8 + (Izz*q3(t)*q4(t)^2*w1(t)^2)/8 + (Izz*q2(t)^2*q3(t)*w3(t)^2)/8 + (Izz*q3(t)*q4(t)^2*w3(t)^2)/8 - (Ixx*q2(t)^3*w1(t)*w2(t))/8 + (Ixx*q2(t)^3*w2(t)*w3(t))/8 + (Ixx*q4(t)^3*w1(t)*w2(t))/8 + (Ixx*q4(t)^3*w2(t)*w3(t))/8 - (Iyy*q2(t)^3*w2(t)*w3(t))/8\\\r\n - (Iyy*q4(t)^3*w2(t)*w3(t))/8 + (Ixx*q1(t)*q2(t)*q4(t)*w1(t)^2)/4 - (Ixx*q1(t)*q2(t)*q4(t)*w3(t)^2)/4 - (Ixx*q2(t)*q3(t)*q4(t)*w1(t)^2)/4 + (Ixx*q2(t)*q3(t)*q4(t)*w3(t)^2)/4 + (Iyy*q1(t)*q2(t)*q4(t)*w2(t)^2)/4 + (Iyy*q2(t)*q3(t)*q4(t)*w1(t)^2)/2 - (Iyy*q2(t)*q3(t)*q4(t)*w2(t)^2)/4 - (Izz*q1(t)*q2(t)*q4(t)*w1(t)^2)/4 + (Izz*q1(t)*q2(t)*q4(t)*w3(t)^2)/4 - (Izz*q2(t)*q3(t)*q4(t)*w1(t)^2)/4 + (Izz*q2(t)*q3(t)*q4(t)*w3(t)^2)/4 + (Ixx*q1(t)^2*q2(t)*w1(t)*w2(t))/4 + (Ixx*q1(t)*q2(t)^2*w1(t)*w3(t))/4 - (Ixx*q1(t)^2*q2(t)*w2(t)*w3(t))/4 - (Ixx*q1(t)^2*q4(t)*w1(t)*w2(t))/4 - (Ixx*q1(t)*q4(t)^2*w1(t)*w3(t))/4 - (Ixx*q2(t)*q4(t)^2*w1(t)*w2(t))/8 - (Ixx*q2(t)^2*q3(t)*w1(t)*w3(t))/4 + (Ixx*q2(t)^2*q4(t)*w1(t)*w2(t))/8 - (Ixx*q1(t)^2*q4(t)*w2(t)*w3(t))/4 + (Ixx*q2(t)*q4(t)^2*w2(t)*w3(t))/8 + (Ixx*q3(t)*q4(t)^2*w1(t)*w3(t))/4 + (Ixx*q2(t)^2*q4(t)*w2(t)*w3(t))/8 - (Iyy*q1(t)^2*q2(t)*w1(t)*w2(t))/8 - (3*Iyy*q2(t)*q3(t)^2*w1(t)*w2(t))/8 + (Iyy*q1(t)^2*q4(t)*w1(t)*w2(t))/8 + (Iyy*q2(t)*q4(t)^2*w1(t)*w2(\\\r\nt))/4 + (Iyy*q2(t)^2*q3(t)*w1(t)*w3(t))/4 - (Iyy*q2(t)^2*q4(t)*w1(t)*w2(t))/4 + (3*Iyy*q3(t)^2*q4(t)*w1(t)*w2(t))/8 + (Iyy*q2(t)*q4(t)^2*w2(t)*w3(t))/8 - (Iyy*q3(t)*q4(t)^2*w1(t)*w3(t))/4 + (Iyy*q2(t)^2*q4(t)*w2(t)*w3(t))/8 - (Izz*q1(t)^2*q2(t)*w1(t)*w2(t))/8 - (Izz*q1(t)*q2(t)^2*w1(t)*w3(t))/4 + (3*Izz*q2(t)*q3(t)^2*w1(t)*w2(t))/8 + (Izz*q1(t)^2*q2(t)*w2(t)*w3(t))/8 + (Izz*q1(t)^2*q4(t)*w1(t)*w2(t))/8 + (Izz*q1(t)*q4(t)^2*w1(t)*w3(t))/4 - (Izz*q2(t)^2*q3(t)*w1(t)*w3(t))/4 - (3*Izz*q2(t)*q3(t)^2*w2(t)*w3(t))/8 + (Izz*q1(t)^2*q4(t)*w2(t)*w3(t))/8 - (3*Izz*q3(t)^2*q4(t)*w1(t)*w2(t))/8 + (Izz*q3(t)*q4(t)^2*w1(t)*w3(t))/4 - (3*Izz*q3(t)^2*q4(t)*w2(t)*w3(t))/8 - (Ixx*q1(t)*q2(t)*q3(t)*w1(t)*w2(t))/2 + (Ixx*q1(t)*q2(t)*q3(t)*w2(t)*w3(t))/2 + (Ixx*q1(t)*q3(t)*q4(t)*w1(t)*w2(t))/2 + (Ixx*q1(t)*q3(t)*q4(t)*w2(t)*w3(t))/2 + (Iyy*q1(t)*q2(t)*q3(t)*w1(t)*w2(t))/4 - (Iyy*q1(t)*q3(t)*q4(t)*w1(t)*w2(t))/4 + (Izz*q1(t)*q2(t)*q3(t)*w1(t)*w2(t))/4 - (Izz*q1(t)*q2(t)*q3(t)*w2(t)*w3(t))/4 - (Izz*q1(t)*q3\\\r\n(t)*q4(t)*w1(t)*w2(t))/4 - (Izz*q1(t)*q3(t)*q4(t)*w2(t)*w3(t))/4, (Ixx*q4(t)^3*w2(t)^2)/4 + (Iyy*q4(t)^3*w3(t)^2)/4 - (Ixx*q1(t)^2*q2(t)*w1(t)^2)/8 - (Ixx*q2(t)*q3(t)^2*w1(t)^2)/8 + (Ixx*q1(t)^2*q2(t)*w3(t)^2)/8 + (Ixx*q1(t)^2*q4(t)*w1(t)^2)/8 + (Ixx*q2(t)*q3(t)^2*w3(t)^2)/8 + (Ixx*q1(t)^2*q4(t)*w3(t)^2)/8 + (Ixx*q2(t)^2*q4(t)*w2(t)^2)/4 + (Ixx*q3(t)^2*q4(t)*w1(t)^2)/8 + (Ixx*q3(t)^2*q4(t)*w3(t)^2)/8 + (Iyy*q1(t)^2*q2(t)*w1(t)^2)/4 - (Iyy*q1(t)^2*q2(t)*w2(t)^2)/8 + (Iyy*q2(t)*q3(t)^2*w1(t)^2)/4 - (Iyy*q2(t)*q3(t)^2*w2(t)^2)/8 + (Iyy*q1(t)^2*q4(t)*w2(t)^2)/8 + (Iyy*q2(t)^2*q4(t)*w1(t)^2)/2 - (Iyy*q2(t)^2*q4(t)*w3(t)^2)/4 + (Iyy*q3(t)^2*q4(t)*w2(t)^2)/8 - (Izz*q1(t)^2*q2(t)*w1(t)^2)/8 - (Izz*q2(t)*q3(t)^2*w1(t)^2)/8 + (Izz*q1(t)^2*q2(t)*w3(t)^2)/8 + (Izz*q1(t)^2*q4(t)*w1(t)^2)/8 + (Izz*q2(t)*q3(t)^2*w3(t)^2)/8 + (Izz*q1(t)^2*q4(t)*w3(t)^2)/8 + (Izz*q3(t)^2*q4(t)*w1(t)^2)/8 + (Izz*q3(t)^2*q4(t)*w3(t)^2)/8 - (Iyy*q1(t)^3*w1(t)*w2(t))/8 + (Iyy*q2(t)^3*w1(t)*w3(t))/4 + (Iyy*q3(t)^3*w1(t)*w2(t))/8 + (Izz*q1(t)^3*w1(t)*w2(t))/8 + (Izz*q1(t)^3*w2(t)*w3(t))/8\\\r\n - (Izz*q3(t)^3*w1(t)*w2(t))/8 - (Izz*q3(t)^3*w2(t)*w3(t))/8 + (Ixx*q1(t)*q2(t)*q3(t)*w1(t)^2)/4 - (Ixx*q1(t)*q2(t)*q3(t)*w3(t)^2)/4 - (Ixx*q1(t)*q3(t)*q4(t)*w1(t)^2)/4 + (Ixx*q1(t)*q3(t)*q4(t)*w2(t)^2)/2 - (Ixx*q1(t)*q3(t)*q4(t)*w3(t)^2)/4 + (Iyy*q1(t)*q2(t)*q3(t)*w2(t)^2)/4 - (Iyy*q1(t)*q3(t)*q4(t)*w2(t)^2)/4 - (Izz*q1(t)*q2(t)*q3(t)*w1(t)^2)/4 + (Izz*q1(t)*q2(t)*q3(t)*w3(t)^2)/4 + (Izz*q1(t)*q3(t)*q4(t)*w1(t)^2)/4 + (Izz*q1(t)*q3(t)*q4(t)*w3(t)^2)/4 - (Ixx*q1(t)*q2(t)^2*w1(t)*w2(t))/8 + (Ixx*q1(t)*q3(t)^2*w1(t)*w2(t))/4 - (Ixx*q1(t)^2*q3(t)*w1(t)*w2(t))/4 - (Ixx*q1(t)*q2(t)^2*w2(t)*w3(t))/8 - (3*Ixx*q1(t)*q4(t)^2*w1(t)*w2(t))/8 + (Ixx*q2(t)^2*q3(t)*w1(t)*w2(t))/8 + (Ixx*q1(t)*q3(t)^2*w2(t)*w3(t))/4 - (Ixx*q1(t)^2*q3(t)*w2(t)*w3(t))/4 + (Ixx*q1(t)^2*q4(t)*w1(t)*w3(t))/4 - (3*Ixx*q1(t)*q4(t)^2*w2(t)*w3(t))/8 + (3*Ixx*q3(t)*q4(t)^2*w1(t)*w2(t))/8 + (Ixx*q2(t)^2*q3(t)*w2(t)*w3(t))/8 + (Ixx*q3(t)^2*q4(t)*w1(t)*w3(t))/4 + (3*Ixx*q3(t)*q4(t)^2*w2(t)*w3(t))/8 + (Iyy*q1(t)*q2(t)^2*w1(t)*w2(\\\r\nt))/4 - (Iyy*q1(t)*q3(t)^2*w1(t)*w2(t))/8 + (Iyy*q1(t)^2*q3(t)*w1(t)*w2(t))/8 - (Iyy*q1(t)*q2(t)^2*w2(t)*w3(t))/8 - (Iyy*q2(t)^2*q3(t)*w1(t)*w2(t))/4 - (Iyy*q1(t)^2*q4(t)*w1(t)*w3(t))/4 + (3*Iyy*q1(t)*q4(t)^2*w2(t)*w3(t))/8 - (3*Iyy*q2(t)*q4(t)^2*w1(t)*w3(t))/4 + (Iyy*q2(t)^2*q3(t)*w2(t)*w3(t))/8 - (Iyy*q3(t)^2*q4(t)*w1(t)*w3(t))/4 - (3*Iyy*q3(t)*q4(t)^2*w2(t)*w3(t))/8 - (Izz*q1(t)*q3(t)^2*w1(t)*w2(t))/8 + (Izz*q1(t)^2*q3(t)*w1(t)*w2(t))/8 - (Izz*q1(t)*q3(t)^2*w2(t)*w3(t))/8 + (Izz*q1(t)^2*q3(t)*w2(t)*w3(t))/8 + (Izz*q1(t)^2*q4(t)*w1(t)*w3(t))/4 + (Izz*q3(t)^2*q4(t)*w1(t)*w3(t))/4 + (Ixx*q1(t)*q2(t)*q4(t)*w1(t)*w2(t))/4 - (Ixx*q1(t)*q2(t)*q4(t)*w2(t)*w3(t))/4 - (Ixx*q1(t)*q3(t)*q4(t)*w1(t)*w3(t))/2 - (Ixx*q2(t)*q3(t)*q4(t)*w1(t)*w2(t))/4 + (Ixx*q2(t)*q3(t)*q4(t)*w2(t)*w3(t))/4 - (Iyy*q1(t)*q2(t)*q4(t)*w1(t)*w2(t))/2 - (Iyy*q1(t)*q2(t)*q4(t)*w2(t)*w3(t))/4 + (Iyy*q2(t)*q3(t)*q4(t)*w1(t)*w2(t))/2 + (Iyy*q2(t)*q3(t)*q4(t)*w2(t)*w3(t))/4 + (Izz*q1(t)*q3(t)*q4(t)*w1(t)*w3(t))/2]



q1=q(1);
q2=q(2);
q3=q(3);
q4=q(4);
Ixx = 0.5;
Iyy = Ixx;
Izz = 2;
% coder.extrinsic('qdottranJqdot_qdot');
% result = qdottranJqdot_qdot(J,q_dot,q1,q2,q3,q4);
%=[q(1);q(2);q(3);q(4)]

diff_q1=[           0,             -(Izz*q2)/4,             -(Iyy*q3)/4,             -(Ixx*q4)/4;
    -(Izz*q2)/4,              (Izz*q1)/2, (Iyy*q4)/4 - (Izz*q4)/4, (Izz*q3)/4 - (Ixx*q3)/4;
    -(Iyy*q3)/4, (Iyy*q4)/4 - (Izz*q4)/4,              (Iyy*q1)/2, (Ixx*q2)/4 - (Iyy*q2)/4;
    -(Ixx*q4)/4, (Izz*q3)/4 - (Ixx*q3)/4, (Ixx*q2)/4 - (Iyy*q2)/4,              (Ixx*q1)/2];
diff_q2=[              (Izz*q2)/2, -(Izz*q1)/4, (Izz*q4)/4 - (Ixx*q4)/4, (Iyy*q3)/4 - (Izz*q3)/4;
    -(Izz*q1)/4,           0,             -(Ixx*q3)/4,             -(Iyy*q4)/4;
    (Izz*q4)/4 - (Ixx*q4)/4, -(Ixx*q3)/4,              (Ixx*q2)/2, (Ixx*q1)/4 - (Iyy*q1)/4;
    (Iyy*q3)/4 - (Izz*q3)/4, -(Iyy*q4)/4, (Ixx*q1)/4 - (Iyy*q1)/4,              (Iyy*q2)/2];
diff_q3=[              (Iyy*q3)/2, (Ixx*q4)/4 - (Iyy*q4)/4, -(Iyy*q1)/4, (Iyy*q2)/4 - (Izz*q2)/4;
    (Ixx*q4)/4 - (Iyy*q4)/4,              (Ixx*q3)/2, -(Ixx*q2)/4, (Izz*q1)/4 - (Ixx*q1)/4;
    -(Iyy*q1)/4,             -(Ixx*q2)/4,           0,             -(Izz*q4)/4;
    (Iyy*q2)/4 - (Izz*q2)/4, (Izz*q1)/4 - (Ixx*q1)/4, -(Izz*q4)/4,              (Izz*q3)/2];
diff_q4=[              (Ixx*q4)/2, (Ixx*q3)/4 - (Iyy*q3)/4, (Izz*q2)/4 - (Ixx*q2)/4, -(Ixx*q1)/4;
    (Ixx*q3)/4 - (Iyy*q3)/4,              (Iyy*q4)/2, (Iyy*q1)/4 - (Izz*q1)/4, -(Iyy*q2)/4;
    (Izz*q2)/4 - (Ixx*q2)/4, (Iyy*q1)/4 - (Izz*q1)/4,              (Izz*q4)/2, -(Izz*q3)/4;
    -(Ixx*q1)/4,             -(Iyy*q2)/4,             -(Izz*q3)/4,           0];

result = 8*[q_dot.'*diff_q1*q_dot;
          q_dot.'*diff_q2*q_dot;
          q_dot.'*diff_q3*q_dot;
          q_dot.'*diff_q4*q_dot];
% result = 1/2*[q_dot.'*diff(J,q1)*q_dot;
%           q_dot.'*diff(J,q2)*q_dot;
%           q_dot.'*diff(J,q3)*q_dot;
%           q_dot.'*diff(J,q4)*q_dot];

== matlab function Motion Equations from Jan Krieglstein/MATLAB Function ==
  data: q input double; R output double
function R = Quat2R(q)
% compute R from quaternion input

R = [q(1)^2 - q(2)^2 - q(3)^2 + q(4)^2,  2*(q(1)*q(2) - q(3)*q(4)),          2*(q(1)*q(3) + q(2)*q(4));
     2*(q(1)*q(2) + q(3)*q(4)),         -q(1)^2 + q(2)^2 - q(3)^2 + q(4)^2,  2*(q(2)*q(3) - q(1)*q(4));
     2*(q(1)*q(3) - q(2)*q(4)),          2*(q(2)*q(3) + q(1)*q(4)),         -q(1)^2 - q(2)^2 + q(3)^2 + q(4)^2];

== matlab function Motion Equations from Jan Krieglstein/MATLAB Function1 ==
  data: w input double; Q output double
function Q = omegaSkew(w)
%#codegen

Q = [0 w(3) -w(2) w(1);
    -w(3) 0 w(1) w(2);
    w(2) -w(1) 0 w(3);
    -w(1) -w(2) -w(3) 0];

== matlab function Motion Equations from Jan Krieglstein/MATLAB Function3 ==
  data: I input double; I_inv output double
function I_inv = inverse(I)

I_inv = inv(I);

== matlab function Motion Equations from Jan Krieglstein/MATLAB Function5 ==
  data: omega input double; w_x output double
function w_x = omegaSkew3D(omega)

w_x = [0 -omega(3) omega(2);
        omega(3) 0 -omega(1);
        -omega(2) omega(1) 0];

== matlab function Motion Equations, p_I3/MATLAB Function15 ==
  data: I input double; I_inv output double
function I_inv = inverse(I)

I_inv = inv(I);

== matlab function Motion Equations, p_I3/MATLAB Function16 ==
  data: omega input double; w_x output double
function w_x = omegaSkew3D(omega)

w_x = [0 -omega(3) omega(2);
        omega(3) 0 -omega(1);
        -omega(2) omega(1) 0];

== matlab function state estimation/MATLAB Function1 ==
  data: R input double; eul output double
function eul = DCM2Euler(R)

%Roll
phi = atan2d(R(3,2),R(3,3));

%Pitch
psi = atan2d(-R(3,1),sqrt(R(1,1)^2 + R(2,1)^2));

%Yaw
gamma = atan2d(R(2,1),R(1,1));

eul=[phi;psi;gamma];

== matlab function state estimation/MATLAB Function ==
  data: rpy input double; R output double
function R = Euler2DCM(rpy)
alpha = rpy(1);
beta = rpy(2);
gamma = rpy(3);

cg = cosd(gamma);
cb = cosd(beta);
sg = sind(gamma);
sb = sind(beta);
sa = sind(alpha);
ca = cosd(alpha);

R = [cg*cb, cg*sb*sa-sg*ca, cg*sb*ca+sg*sa;
    sg*cb, sg*sb*sa+cg*ca, sg*sb*ca-cg*sa;
    -sb, cb*sa, cb*ca];

== matlab function DC Motor Dynamics incl. FF/MATLAB Function4 ==
  data: u input double; y output double
function y = fcn(u)

y = sqrt(abs(u))*sign(u);

== matlab function control allocation/omega_square to omega ==
  data: u input double; y output double
function y = square2omega(u)

y = sqrt(abs(u)).*sign(u);

== matlab function control effectiveness model/omega to omega_square ==
  data: u input double; y output double
function y = omega2square(u)

y = u.^2.*sign(u);
